simulink model "aaaaaa"  (R2018b)
settings: Solver=VariableStepAuto  StartTime=0.0  StopTime=30  MaxStep=0.01  RelTol=1e-3
values from neighbouring files (symbols this model uses):
  A = [0 1; 4 0]    [snatch3.m]    (also in snatch4.m; snatch5.m; snatch6.m)
  B = [1; 1]    [snatch3.m]    (also in snatch4.m; snatch5.m; snatch6.m)
  C = [3 0]    [snatch3.m]    (also in snatch4.m; snatch5.m; snatch6.m)
  K = inv(R)*transpose(B)*P    [snatch3.m]    (also in snatch4.m = [k1Sol(2) k2Sol(2)]; snatch5.m; snatch6.m = [k1Sol(2) k2Sol(2)])
  L = [k1Sol; k2Sol]    [snatch4.m]
settings Model: Creator=kekos  LastModifiedBy=kekos

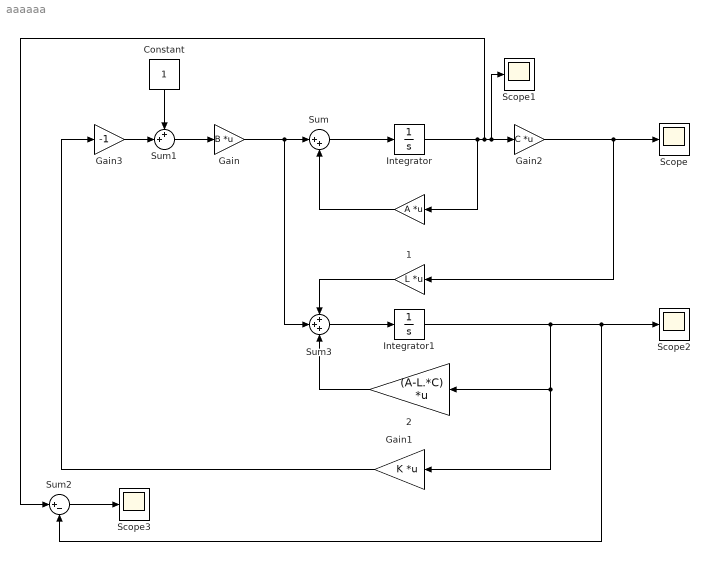
== system aaaaaa ==
  " " : Gain  Gain=A  Multiplication=Matrix(K*u)
  " 1" : Gain  Gain=L  Multiplication=Matrix(K*u)
  " 2" : Gain  Gain=(A-L.*C)  Multiplication=Matrix(K*u)
  Constant : Constant
  Gain : Gain  Gain=B  Multiplication=Matrix(K*u)
  Gain1 : Gain  Gain=K  Multiplication=Matrix(K*u)
  Gain2 : Gain  Gain=C  Multiplication=Matrix(K*u)
  Gain3 : Gain  Gain=-1
  Integrator : Integrator  InitialCondition=[1; 1]
  Integrator1 : Integrator
  Scope{,1..3} (4 alike) : Scope
  Sum : Sum  Inputs=|++
  Sum1 : Sum  Inputs=++|
  Sum2 : Sum  Inputs=|+-
  Sum3 : Sum  Inputs=+++
  wires:
  Gain/1 -> Sum3/2, Sum/1
  " 2"/1 -> Sum3/3
  Gain2/1 -> " 1"/1, Scope/1
  Integrator1/1 -> Sum2/2, Scope2/1, Gain1/1, " 2"/1
  " "/1 -> Sum/2
  Gain3/1 -> Sum1/2
  Integrator/1 -> Sum2/1, Scope1/1, Gain2/1, " "/1
  Gain1/1 -> Gain3/1
  Sum1/1 -> Gain/1
  Constant/1 -> Sum1/1
  " 1"/1 -> Sum3/1
  Sum3/1 -> Integrator1/1
  Sum/1 -> Integrator/1
  Sum2/1 -> Scope3/1
